simulink model "inv_pen"  (R2014a)
settings: Solver=ode45  SolverMode=SingleTasking  StartTime=0.0  StopTime=100  RelTol=1e-3
values from neighbouring files (symbols this model uses):
  A = load('../A.csv')    [probofminobj.m]    (also in sim_inv.m = zeros(n1+m1,n1+m1); sugarmill.m = zeros(n1+m1,n1+m1); testCMPC.m = zeros(n1+m1,n1+m1))
  B = load('../B.csv')    [probofminobj.m]    (also in sim_inv.m = zeros(n1+m1,n_in); sugarmill.m = zeros(n1+m1,n_in); testCMPC.m = zeros(n1+m1,n_in))
  C = zeros(m1,n1+m1)    [sim_inv.m]    (also in sugarmill.m; testCMPC.m)
undefined symbols (not defined in the file or in its folder): D, x0
libraries: mpclib x1
settings Model: ExtModeTrigMode=oneshot  ExtModeArmWhenConnect=off  Creator=jowen  LastModifiedBy=ares
settings DataIOCC: LimitDataPoints=off  SignalLoggingSaveFormat=ModelDataLogs  SignalLoggingName=sigsOut
settings OptimizationCC: BooleanDataType=off  ExpressionDepthLimit=2147483647  InitFltsAndDblsToZero=on
settings DebuggingCC: SaveWithParameterizedLinksMsg=none  UnderspecifiedInitializationDetection=Classic  CheckExecutionContextPreStartOutputMsg=on  CheckExecutionContextRuntimeOutputMsg=on  SignalResolutionControl=TryResolveAllWithWarning  SolverPrmCheckMsg=none  MultiTaskDSMMsg=warning  MultiTaskCondExecSysMsg=none  IntegerOverflowMsg=none  FcnCallInpInsideContextMsg=UseLocalSettings  StateNameClashWarn=warning
settings HardwareCC: TargetUnknown=on
settings RTWCC: IncludeERTFirstTime=on
settings GRTTargetCC: TargetFcnLib=ansi_tfl_tmw.mat  CombineOutputUpdateFcns=off  GRTInterface=on

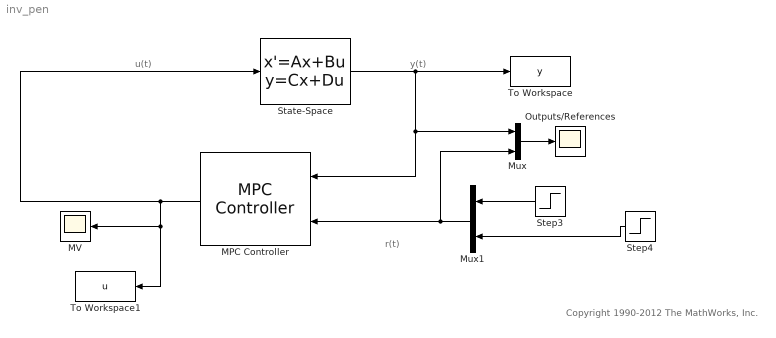
== system inv_pen ==
  note: u(t)
  note: y(t)
  note: r(t)
  note: Copyright 1990-2012 The MathWorks, Inc.
  MPC Controller : mpclib/MPC Controller  mpcobj=mpcafti  x0=[]  md_inport=off  mv_inport=off  lims_inport=off  switch_inport=off  ywt_inport=off  duwt_inport=off  rhoeps_inport=off  cost_outport=off  return_sequence=off  return_qpstatus=off  is_multiple=0  enable_value=0  n_mv=1  n_mo=2  n_md=0  n_ts=0.02  is_designfromscratch=0  BlockDataType=double  SampleTimeInherited=off  ref_from_ws=off  ref_signal_name=[]  ref_preview=on  md_from_ws=off  md_signal_name=[]  md_preview=on  from_project=off  project_file=MPCtask.mat
  MV : Scope
      settings: TimeRange=2  YMin=-20  YMax=30  DataFormat=Structure
  Mux : Mux  Inputs=2
  Mux1 : Mux  Inputs=2
  Outputs/References : Scope
      settings: TimeRange=2  YMax=15  DataFormat=Structure
  State-Space : StateSpace  A=A  B=B  C=C  D=D  X0=x0
  Step3 : Step  Time=0  After=0  SampleTime=0
  Step4 : Step  Time=0  After=0  SampleTime=0
  To Workspace : ToWorkspace  VariableName=y  SampleTime=-1
  To Workspace1 : ToWorkspace  VariableName=u  SampleTime=-1
  wires:
  State-Space/1 -> To Workspace/1, Mux/1, MPC Controller/1
  Mux/1 -> Outputs/References/1
  MPC Controller/1 -> MV/1, To Workspace1/1, State-Space/1
  Step3/1 -> Mux1/1
  Step4/1 -> Mux1/2
  Mux1/1 -> Mux/2, MPC Controller/2
